simulink model "Grp43_Model2"  (R2023a)
settings: Solver=VariableStepAuto  StartTime=0.0  StopTime=10.0  RelTol=1e-3
values from neighbouring files (symbols this model uses):
  den = [1, 0, -30.17, 0, 0]    [Grp43_part2_code.m]
  denC = [1, q0]    [Grp43_part2_code.m]
  g = 9.8    [Grp43_Code.m]    (also in Grp43_part2_code.m = 9.81; e01 2.m; grp43_asgn2_2.m)
  l = 0.36    [Grp43_Code.m]    (also in Grp43_part2_code.m; e01 2.m; grp43_asgn2_2.m)
  m = 0.26    [Grp43_Code.m]    (also in Grp43_part2_code.m; e01 2.m; grp43_asgn2_2.m)
  M = 2.4    [Grp43_Code.m]    (also in Grp43_part2_code.m; e01 2.m; grp43_asgn2_2.m)
  num1 = [a0, a1]    [Grp43_part2_code.m]
  num2 = [p0, p1]    [Grp43_part2_code.m]
  numX = [0.4167, 0, -12.41]    [Grp43_part2_code.m]
  numY = [-0.15, 0, 0]    [Grp43_part2_code.m]
settings Model: Creator=Anirvan Krishna  LastModifiedBy=Anirvan Krishna

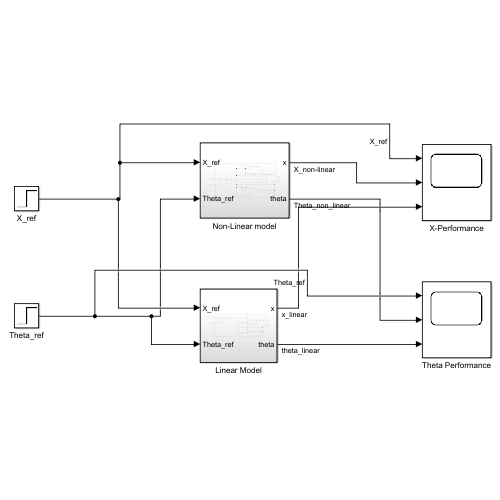
[thumbnail: Simulink's stored preview of the top-level diagram]
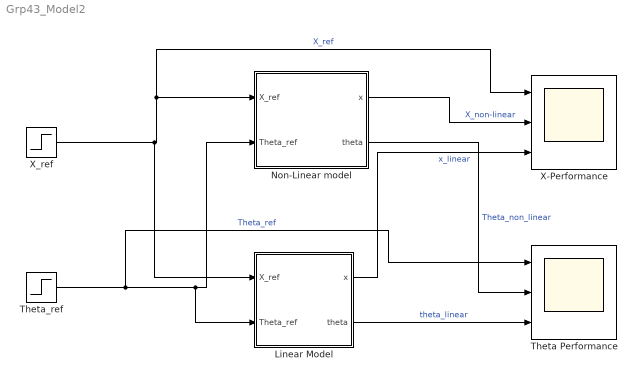
== system Grp43_Model2 ==
  Linear Model : Subsystem
  Non-Linear model : Subsystem
  Theta Performance : Scope  NumInputPorts=3
  Theta_ref : Step  Time=0.1  SampleTime=0
  X-Performance : Scope  NumInputPorts=3
  X_ref : Step  Time=0.1  SampleTime=0
  wires:
  Non-Linear model/1(x) -> X-Performance/2  "X_non-linear"
  X_ref/1 -> Linear Model/1(X_ref), X-Performance/1, Non-Linear model/1(X_ref)  "X_ref"
  Theta_ref/1 -> Theta Performance/1, Linear Model/2(Theta_ref), Non-Linear model/2(Theta_ref)  "Theta_ref"
  Non-Linear model/2(theta) -> Theta Performance/2  "Theta_non_linear"
  Linear Model/2(theta) -> Theta Performance/3  "theta_linear"
  Linear Model/1(x) -> X-Performance/3  "x_linear"

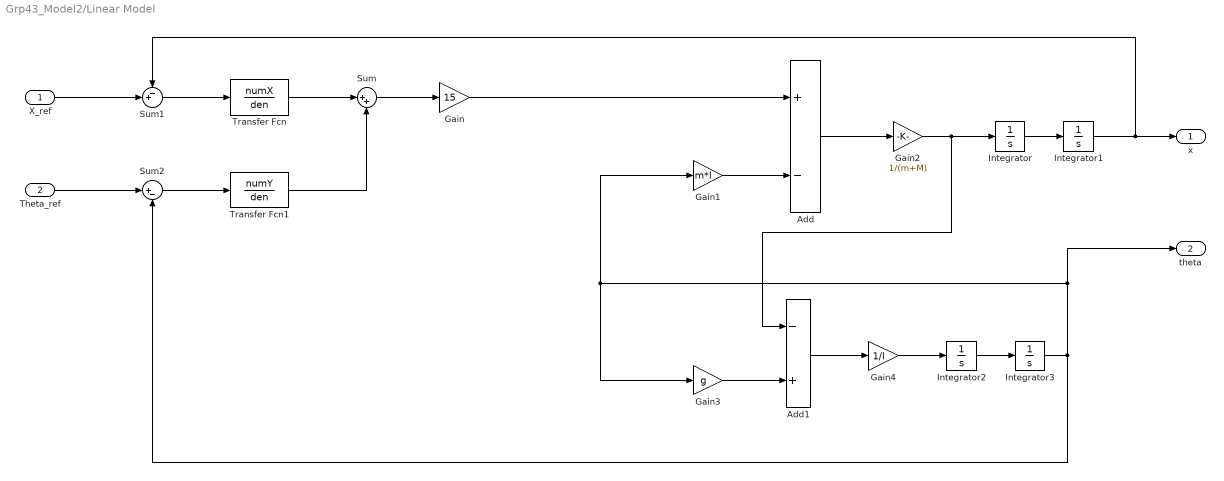
== system Grp43_Model2/Linear Model ==
  X_ref : Inport
  Theta_ref : Inport  Port=2
  Add : Sum  Inputs=+-
  Add1 : Sum  Inputs=-+
  Gain : Gain  Gain=15
  Gain1 : Gain  Gain=m*l
  Gain2 : Gain  Gain=1/(m+M)
  Gain3 : Gain  Gain=g
  Gain4 : Gain  Gain=1/l
  Integrator{,1..3} (4 alike) : Integrator
  Sum : Sum  Inputs=|++
  Sum1 : Sum  Inputs=-+|
  Sum2 : Sum  Inputs=|+-
  Transfer Fcn : TransferFcn  Numerator=numX  Denominator=den  ContinuousStateAttributes='c1'
  Transfer Fcn1 : TransferFcn  Numerator=numY  Denominator=den  ContinuousStateAttributes='c2'
  x : Outport
  theta : Outport  Port=2
  wires:
  Sum2/1 -> Transfer Fcn1/1
  Transfer Fcn/1 -> Sum/1
  Transfer Fcn1/1 -> Sum/2
  Sum1/1 -> Transfer Fcn/1
  Sum/1 -> Gain/1
  X_ref/1 -> Sum1/2
  Theta_ref/1 -> Sum2/1
  Add/1 -> Gain2/1
  Gain4/1 -> Integrator2/1
  Integrator1/1 -> x/1, Sum1/1
  Gain2/1 -> Add1/1, Integrator/1
  Gain3/1 -> Add1/2
  Gain/1 -> Add/1
  Add1/1 -> Gain4/1
  Integrator/1 -> Integrator1/1
  Integrator3/1 -> theta/1, Gain1/1, Gain3/1, Sum2/2
  Integrator2/1 -> Integrator3/1
  Gain1/1 -> Add/2

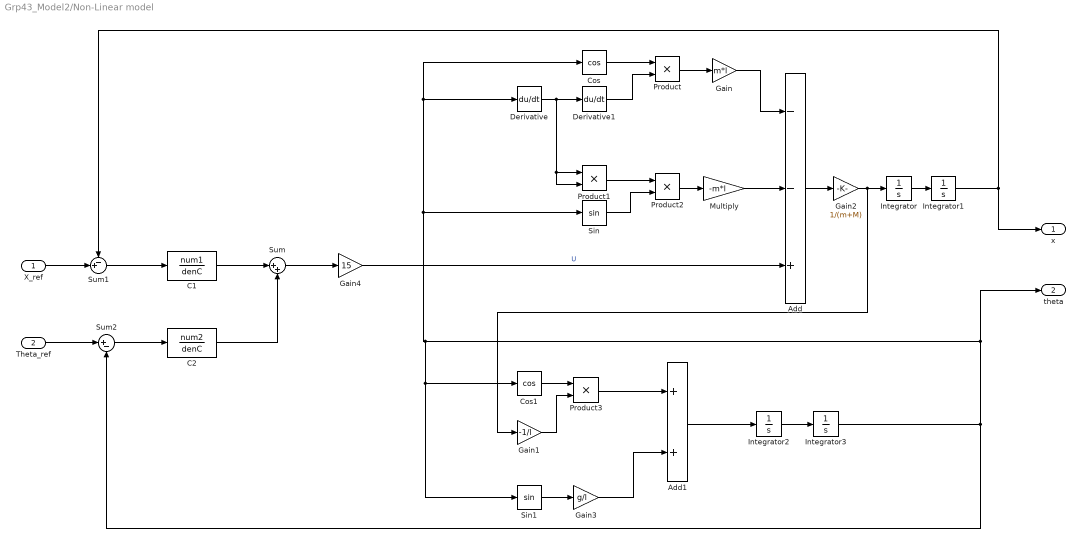
== system Grp43_Model2/Non-Linear model ==
  X_ref : Inport
  Theta_ref : Inport  Port=2
  Add : Sum  Inputs=--+
  Add1 : Sum
  C1 : TransferFcn  Numerator=num1  Denominator=denC  ContinuousStateAttributes='g1'
  C2 : TransferFcn  Numerator=num2  Denominator=denC  ContinuousStateAttributes='g2'
  Cos : Trigonometry  Operator=cos
  Cos1 : Trigonometry  Operator=cos
  Derivative : Derivative
  Derivative1 : Derivative
  Gain : Gain  Gain=m*l
  Gain1 : Gain  Gain=-1/l
  Gain2 : Gain  Gain=1/(m+M)
  Gain3 : Gain  Gain=g/l
  Gain4 : Gain  Gain=15
  Integrator{,1..3} (4 alike) : Integrator
  Multiply : Gain  Gain=-m*l
  Product{,1..3} (4 alike) : Product
  Sin : Trigonometry
  Sin1 : Trigonometry
  Sum : Sum  Inputs=|++
  Sum1 : Sum  Inputs=-+|
  Sum2 : Sum  Inputs=|+-
  x : Outport
  theta : Outport  Port=2
  wires:
  Multiply/1 -> Add/2
  Integrator3/1 -> theta/1, Cos1/1, Sin1/1, Cos/1, Derivative/1, Sin/1, Sum2/2
  Integrator2/1 -> Integrator3/1
  Product1/1 -> Product2/1
  Cos/1 -> Product/1
  Cos1/1 -> Product3/1
  Sin1/1 -> Gain3/1
  Gain/1 -> Add/1
  Add/1 -> Gain2/1
  Add1/1 -> Integrator2/1
  Derivative/1 -> Product1/1, Product1/2, Derivative1/1
  Gain3/1 -> Add1/2
  Product2/1 -> Multiply/1
  Derivative1/1 -> Product/2
  Product3/1 -> Add1/1
  Sin/1 -> Product2/2
  Gain1/1 -> Product3/2
  Gain2/1 -> Gain1/1, Integrator/1
  Product/1 -> Gain/1
  Integrator/1 -> Integrator1/1
  Integrator1/1 -> x/1, Sum1/1
  Sum/1 -> Gain4/1
  C1/1 -> Sum/1
  C2/1 -> Sum/2
  Gain4/1 -> Add/3  "U"
  Theta_ref/1 -> Sum2/1
  Sum2/1 -> C2/1
  Sum1/1 -> C1/1
  X_ref/1 -> Sum1/2
